simulink model "AnalyseIMUData_LSM9DS1"  (R2022a)
settings: Solver=FixedStepAuto  StartTime=0.0  StopTime=inf  RelTol=1e-3  EnableMultiTasking=on
libraries: arduinosensorlib x1, arduinolib x1
settings Model: ExtModeTrigDuration=2  Creator=The MathWorks, Inc.  LastModifiedBy=cwpan
settings SolverCC: MaxZcPerStep=1
settings OptimizationCC: EnhancedBackFolding=on  PassReuseOutputArgsAs=Individual arguments  ZeroExternalMemoryAtStartup=off  ZeroInternalMemoryAtStartup=off  MaxStackSize=64  OptimizeBlockOrder=speed  DifferentSizesBufferReuse=on  OptimizationCustomize=off  EfficientTunableParamExpr=on
settings DebuggingCC: ParameterPrecisionLossMsg=none  ParameterTunabilityLossMsg=error  UnconnectedInputMsg=warning  UnconnectedOutputMsg=warning  UnconnectedLineMsg=warning
settings HardwareCC: ProdBitPerInt=16  ProdBitPerPointer=16  ProdBitPerSizeT=16  ProdBitPerPtrDiffT=16  ProdLargestAtomicFloat=None  ProdWordSize=8  ProdHWDeviceType=Atmel->AVR  UseEmbeddedCoderFeatures=off  UseSimulinkCoderFeatures=off
settings SFSimCC: MATLABDynamicMemAlloc=off
settings RTWCC: SystemTargetFile=ert.tlc  HardwareBoard=Arduino Uno  TemplateMakefile=ert_default_tmf  Toolchain=Arduino AVR  BuildConfiguration=Faster Runs  DLArmComputeVersion=19.05
settings CodeAppCC: ForceParamTrailComments=on  IgnoreCustomStorageClasses=off  OperatorAnnotations=on  SimulinkDataObjDesc=on  SFDataObjDesc=on  InsertBlockDesc=on
settings ERTTargetCC: SupportContinuousTime=on  SupportNonInlinedSFcns=on  SupportVariableSizeSignals=on  ExtModeTransport=3  ExtModeStaticAlloc=on  ExtModeStaticAllocSize=250  ExtModeMexFile=ext_xcp  ExtModeIntrfLevel=Level2 - Open

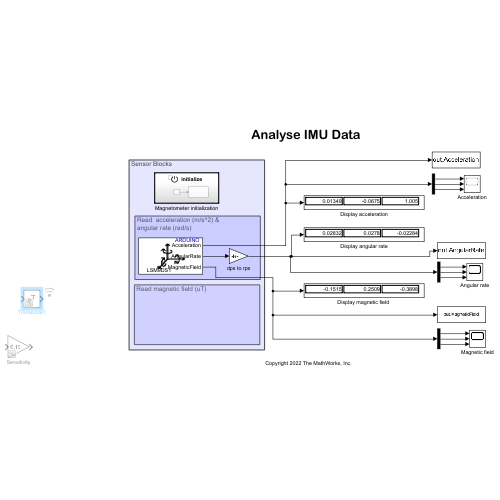
[thumbnail: Simulink's stored preview of the top-level diagram]
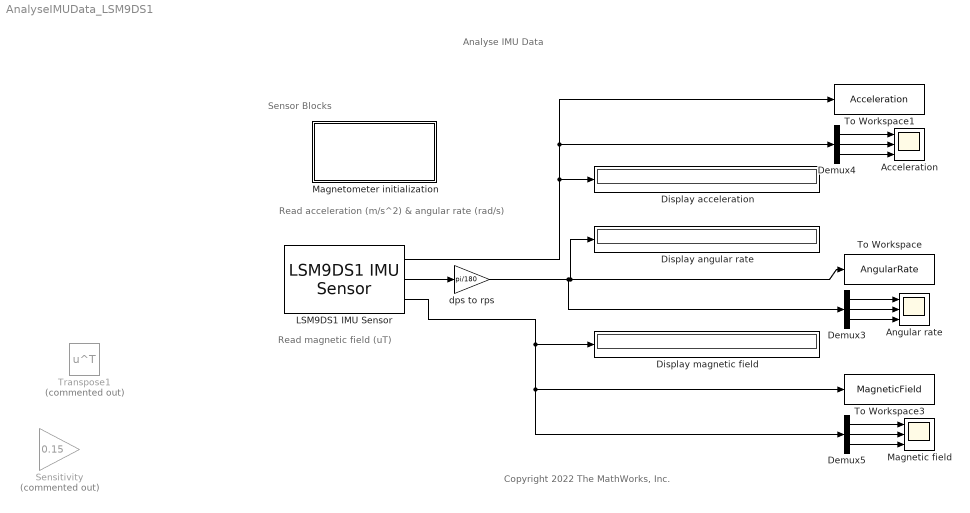
== system AnalyseIMUData_LSM9DS1 ==
  note: Read  acceleration (m/s^2) &
      | angular rate (rad/s)
  note: Read magnetic field (uT)
  note: Sensor Blocks
  note: Copyright 2022 The MathWorks, Inc.
  note: Analyse IMU Data
  Acceleration : Scope  NumInputPorts=3
  Angular rate : Scope  NumInputPorts=3
  Demux3 : Demux  Outputs=3
  Demux4 : Demux  Outputs=3
  Demux5 : Demux  Outputs=3
  Display acceleration : Display
  Display angular rate : Display
  "Display magnetic field " : Display
  LSM9DS1 IMU Sensor : arduinosensorlib/LSM9DS1 IMU Sensor  AccelandGyroAddress=0x6B  MagnetometerAddress=0x1E  EnableAccel=on  EnableGyro=on  EnableMag=on  AccelerometerOutputDataRate=119 Hz  AccelerometerFullScaleRange=+/- 2g  AccelerometerBandwidth=50 Hz  GyroscopeOutputDataRate=119 Hz  GyroscopeFullScaleRange=245 dps  GyroscopeBandwidthMode=0  GyroscopeHighPassFilterEnabled=on  GyroscopeHighPassFilterMode=0  MagnetometerOutputDataRate=40 Hz  MagnetometerFullScaleRange=+/- 4 gauss  SampleTime=0.1
      settings: SourceProductBaseCode=ARDUINO
  Magnetic field : Scope  NumInputPorts=3
  Magnetometer initialization : Subsystem  TreatAsAtomicUnit=on
  Sensitivity : Gain  Commented=on  Gain=0.15  OutDataTypeStr=double  LockScale=on
  To Workspace : ToWorkspace  VariableName=AngularRate  SampleTime=-1
      settings: Save2DSignal=2-D array (concatenate along first dimension)
  To Workspace1 : ToWorkspace  VariableName=Acceleration  SampleTime=-1
      settings: Save2DSignal=2-D array (concatenate along first dimension)
  To Workspace3 : ToWorkspace  VariableName=MagneticField  SampleTime=-1
      settings: Save2DSignal=2-D array (concatenate along first dimension)
  Transpose1 : Math  Commented=on  Operator=transpose
  dps to rps : Gain  Gain=pi/180  OutDataTypeStr=double  LockScale=on
  wires:
  Demux4/1 -> Acceleration/1
  Demux4/3 -> Acceleration/3
  Demux4/2 -> Acceleration/2
  Demux5/3 -> Magnetic field/3
  Demux5/2 -> Magnetic field/2
  LSM9DS1 IMU Sensor/1 -> To Workspace1/1, Demux4/1, Display acceleration/1
  Demux5/1 -> Magnetic field/1
  Demux3/1 -> Angular rate/1
  Demux3/2 -> Angular rate/2
  Demux3/3 -> Angular rate/3
  LSM9DS1 IMU Sensor/2 -> dps to rps/1
  dps to rps/1 -> To Workspace/1, Display angular rate/1, Demux3/1
  LSM9DS1 IMU Sensor/3 -> "Display magnetic field "/1, Demux5/1, To Workspace3/1

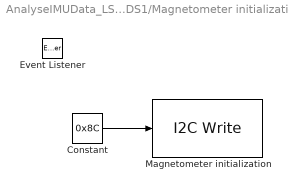
== system AnalyseIMUData_LSM9DS1/Magnetometer initialization ==
  Constant : Constant  Value=0x8C  OutDataTypeStr=uint8
  Event Listener : EventListener  DisableCoverage=on  EventName=reset
  Magnetometer initialization : arduinolib/I2C Write  Priority=1  I2CModule=0  Mode=Master  SlaveAddress=0x1E  SlaveByteOrder=LittleEndian  Direction=Transmitter  RegisterAddressMode=on  RegisterAddress=0x60  SlaveDataType=uint8  DataLength=1  NoAck=off  RepeatedStart=off  OutputStatus=off  blockPlatform=ARDUINO
      settings: SourceProductBaseCode=ARDUINO
  wires:
  Constant/1 -> Magnetometer initialization/1
